simulink model "kestfilt_2048ch_60mhz"  (R2013b)
settings: Solver=FixedStepDiscrete  SolverMode=SingleTasking  StartTime=0.0  StopTime=100.0  FixedStep=0.1  RelTol=1e-3
undefined symbols (not defined in the file): calan_lib, comp_addsub, internal_oor, minmax, misc_lib, nonstop_vacc, pfb_coeff_gen_calc, seq_minmax, xlfda_numerator, xlipgetpartsetting
libraries: xbsIndex_r4 x3129, casper_library_misc x28, xps_library x27, dspsigops x16, casper_library_delays x7, simulink x2
(part 4 of 32)

== system kestfilt_2048ch_60mhz/dec_fir1 ==
  sync_in : Inport
  real1 : Inport  Port=2
  imag1 : Inport  Port=3
  real2 : Inport  Port=4
  imag2 : Inport  Port=5
  real3 : Inport  Port=6
  imag3 : Inport  Port=7
  real4 : Inport  Port=8
  imag4 : Inport  Port=9
  real5 : Inport  Port=10
  imag5 : Inport  Port=11
  real6 : Inport  Port=12
  imag6 : Inport  Port=13
  real7 : Inport  Port=14
  imag7 : Inport  Port=15
  real8 : Inport  Port=16
  imag8 : Inport  Port=17
  convert1 : xbsIndex_r4/Convert  gui_display_data_type=Fixed-point  arith_type="Signed  (2's comp)"  n_bits=8  bin_pt=7  float_type=Single  exp_bits=8  fraction_bits=24  quantization="Round  (unbiased: Even Values)"  overflow=Wrap  en=off  latency=2  dbl_ovrd=off  pipeline=off  block_type=convert
  convert2 : xbsIndex_r4/Convert  gui_display_data_type=Fixed-point  arith_type="Signed  (2's comp)"  n_bits=8  bin_pt=7  float_type=Single  exp_bits=8  fraction_bits=24  quantization="Round  (unbiased: Even Values)"  overflow=Wrap  en=off  latency=2  dbl_ovrd=off  pipeline=off  block_type=convert
  delay : xbsIndex_r4/Delay  rst=off  infoeditControl=Selection of Reset will increase slice count due to use of real FFs and instead of SRLs  en=off  latency=7  dbl_ovrd=off  reg_retiming=off  block_type=delay
  fir_col1 : Subsystem  AncestorBlock=casper_library_downconverter/fir_col  mask(fir_col){n_inputs=8, coeff=[0.00113   0.0022337   0.0028132   0.0028275   0.0023426   0.0015071   0.0005151  -0.0004352], add_latency=1, mult_latency=2, coeff_bit_width=25, coeff_bin_pt=24, first_stage_hdl=on, adder_imp=DSP48}
      mask prompts: n_inputs "Inputs"; coeff "Coefficients"; add_latency "Add latency"; mult_latency "Mult Latency"; coeff_bit_width "Coefficient bit width"; coeff_bin_pt "Coefficient binary point"; first_stage_hdl "Implement first stage of adder trees on output as behavioural HDL"; adder_imp "Adder implementation"
      mask init: same as kestfilt_2048ch_60mhz/dec_fir/fir_col1
      mask Help: eval('xlWeb(''http://casper.berkeley.edu/wiki/Fir_col'')')
      mask TypeOptions adder_imp: Behavioral | Fabric | DSP48
  fir_col10 : Subsystem  AncestorBlock=casper_library_downconverter/fir_col  mask(fir_col){n_inputs=8, coeff=[-0.0058263  -0.0086204   -0.010054  -0.0096853  -0.0073661   -0.003308   0.0019177   0.0074447], add_latency=1, mult_latency=2, coeff_bit_width=25, coeff_bin_pt=24, first_stage_hdl=on, adder_imp=DSP48}
      mask prompts: n_inputs "Inputs"; coeff "Coefficients"; add_latency "Add latency"; mult_latency "Mult Latency"; coeff_bit_width "Coefficient bit width"; coeff_bin_pt "Coefficient binary point"; first_stage_hdl "Implement first stage of adder trees on output as behavioural HDL"; adder_imp "Adder implementation"
      mask init: same as kestfilt_2048ch_60mhz/dec_fir/fir_col1
      mask Help: eval('xlWeb(''http://casper.berkeley.edu/wiki/Fir_col'')')
      mask TypeOptions adder_imp: Behavioral | Fabric | DSP48
  fir_col11 : Subsystem  AncestorBlock=casper_library_downconverter/fir_col  mask(fir_col){n_inputs=8, coeff=[0.0022453   0.0045072   0.0061467   0.0067686   0.0061328   0.0042185   0.0012532  -0.0023042], add_latency=1, mult_latency=2, coeff_bit_width=25, coeff_bin_pt=24, first_stage_hdl=on, adder_imp=DSP48}
      mask prompts: n_inputs "Inputs"; coeff "Coefficients"; add_latency "Add latency"; mult_latency "Mult Latency"; coeff_bit_width "Coefficient bit width"; coeff_bin_pt "Coefficient binary point"; first_stage_hdl "Implement first stage of adder trees on output as behavioural HDL"; adder_imp "Adder implementation"
      mask init: same as kestfilt_2048ch_60mhz/dec_fir/fir_col1
      mask Help: eval('xlWeb(''http://casper.berkeley.edu/wiki/Fir_col'')')
      mask TypeOptions adder_imp: Behavioral | Fabric | DSP48
  fir_col12 : Subsystem  AncestorBlock=casper_library_downconverter/fir_col  mask(fir_col){n_inputs=8, coeff=[-0.00034455  -0.0019414  -0.0033558  -0.0042822  -0.0044754  -0.0038077  -0.0023081 -0.00017465], add_latency=1, mult_latency=2, coeff_bit_width=25, coeff_bin_pt=24, first_stage_hdl=on, adder_imp=DSP48}
      mask prompts: n_inputs "Inputs"; coeff "Coefficients"; add_latency "Add latency"; mult_latency "Mult Latency"; coeff_bit_width "Coefficient bit width"; coeff_bin_pt "Coefficient binary point"; first_stage_hdl "Implement first stage of adder trees on output as behavioural HDL"; adder_imp "Adder implementation"
      mask init: same as kestfilt_2048ch_60mhz/dec_fir/fir_col1
      mask Help: eval('xlWeb(''http://casper.berkeley.edu/wiki/Fir_col'')')
      mask TypeOptions adder_imp: Behavioral | Fabric | DSP48
  fir_col13 : Subsystem  AncestorBlock=casper_library_downconverter/fir_col  mask(fir_col){n_inputs=8, coeff=[-0.0004352   0.0005151   0.0015071   0.0023426   0.0028275   0.0028132   0.0022337     0.00113], add_latency=1, mult_latency=2, coeff_bit_width=25, coeff_bin_pt=24, first_stage_hdl=on, adder_imp=DSP48}
      mask prompts: n_inputs "Inputs"; coeff "Coefficients"; add_latency "Add latency"; mult_latency "Mult Latency"; coeff_bit_width "Coefficient bit width"; coeff_bin_pt "Coefficient binary point"; first_stage_hdl "Implement first stage of adder trees on output as behavioural HDL"; adder_imp "Adder implementation"
      mask init: same as kestfilt_2048ch_60mhz/dec_fir/fir_col1
      mask Help: eval('xlWeb(''http://casper.berkeley.edu/wiki/Fir_col'')')
      mask TypeOptions adder_imp: Behavioral | Fabric | DSP48
  fir_col2 : Subsystem  AncestorBlock=casper_library_downconverter/fir_col  mask(fir_col){n_inputs=8, coeff=[-0.00017465  -0.0023081  -0.0038077  -0.0044754  -0.0042822  -0.0033558  -0.0019414 -0.00034455], add_latency=1, mult_latency=2, coeff_bit_width=25, coeff_bin_pt=24, first_stage_hdl=on, adder_imp=DSP48}
      mask prompts: n_inputs "Inputs"; coeff "Coefficients"; add_latency "Add latency"; mult_latency "Mult Latency"; coeff_bit_width "Coefficient bit width"; coeff_bin_pt "Coefficient binary point"; first_stage_hdl "Implement first stage of adder trees on output as behavioural HDL"; adder_imp "Adder implementation"
      mask init: same as kestfilt_2048ch_60mhz/dec_fir/fir_col1
      mask Help: eval('xlWeb(''http://casper.berkeley.edu/wiki/Fir_col'')')
      mask TypeOptions adder_imp: Behavioral | Fabric | DSP48
  fir_col3 : Subsystem  AncestorBlock=casper_library_downconverter/fir_col  mask(fir_col){n_inputs=8, coeff=[-0.0023042   0.0012532   0.0042185   0.0061328   0.0067686   0.0061467   0.0045072   0.0022453], add_latency=1, mult_latency=2, coeff_bit_width=25, coeff_bin_pt=24, first_stage_hdl=on, adder_imp=DSP48}
      mask prompts: n_inputs "Inputs"; coeff "Coefficients"; add_latency "Add latency"; mult_latency "Mult Latency"; coeff_bit_width "Coefficient bit width"; coeff_bin_pt "Coefficient binary point"; first_stage_hdl "Implement first stage of adder trees on output as behavioural HDL"; adder_imp "Adder implementation"
      mask init: same as kestfilt_2048ch_60mhz/dec_fir/fir_col1
      mask Help: eval('xlWeb(''http://casper.berkeley.edu/wiki/Fir_col'')')
      mask TypeOptions adder_imp: Behavioral | Fabric | DSP48
  fir_col4 : Subsystem  AncestorBlock=casper_library_downconverter/fir_col  mask(fir_col){n_inputs=8, coeff=[0.0074447   0.0019177   -0.003308  -0.0073661  -0.0096853   -0.010054  -0.0086204  -0.0058263], add_latency=1, mult_latency=2, coeff_bit_width=25, coeff_bin_pt=24, first_stage_hdl=on, adder_imp=DSP48}
      mask prompts: n_inputs "Inputs"; coeff "Coefficients"; add_latency "Add latency"; mult_latency "Mult Latency"; coeff_bit_width "Coefficient bit width"; coeff_bin_pt "Coefficient binary point"; first_stage_hdl "Implement first stage of adder trees on output as behavioural HDL"; adder_imp "Adder implementation"
      mask init: same as kestfilt_2048ch_60mhz/dec_fir/fir_col1
      mask Help: eval('xlWeb(''http://casper.berkeley.edu/wiki/Fir_col'')')
      mask TypeOptions adder_imp: Behavioral | Fabric | DSP48
  fir_col5 : Subsystem  AncestorBlock=casper_library_downconverter/fir_col  mask(fir_col){n_inputs=8, coeff=[-0.018838  -0.0098708 -0.00058855   0.0074448     0.01308    0.015703     0.01527    0.012239], add_latency=1, mult_latency=2, coeff_bit_width=25, coeff_bin_pt=24, first_stage_hdl=on, adder_imp=DSP48}
      mask prompts: n_inputs "Inputs"; coeff "Coefficients"; add_latency "Add latency"; mult_latency "Mult Latency"; coeff_bit_width "Coefficient bit width"; coeff_bin_pt "Coefficient binary point"; first_stage_hdl "Implement first stage of adder trees on output as behavioural HDL"; adder_imp "Adder implementation"
      mask init: same as kestfilt_2048ch_60mhz/dec_fir/fir_col1
      mask Help: eval('xlWeb(''http://casper.berkeley.edu/wiki/Fir_col'')')
      mask TypeOptions adder_imp: Behavioral | Fabric | DSP48
  fir_col6 : Subsystem  AncestorBlock=casper_library_downconverter/fir_col  mask(fir_col){n_inputs=8, coeff=[0.065516    0.039865    0.016011  -0.0038951   -0.018338   -0.026596   -0.028772   -0.025715], add_latency=1, mult_latency=2, coeff_bit_width=25, coeff_bin_pt=24, first_stage_hdl=on, adder_imp=DSP48}
      mask prompts: n_inputs "Inputs"; coeff "Coefficients"; add_latency "Add latency"; mult_latency "Mult Latency"; coeff_bit_width "Coefficient bit width"; coeff_bin_pt "Coefficient binary point"; first_stage_hdl "Implement first stage of adder trees on output as behavioural HDL"; adder_imp "Adder implementation"
      mask init: same as kestfilt_2048ch_60mhz/dec_fir/fir_col1
      mask Help: eval('xlWeb(''http://casper.berkeley.edu/wiki/Fir_col'')')
      mask TypeOptions adder_imp: Behavioral | Fabric | DSP48
  fir_col7 : Subsystem  AncestorBlock=casper_library_downconverter/fir_col  mask(fir_col){n_inputs=8, coeff=[0.090423     0.11197     0.12783     0.13623     0.13623     0.12783     0.11197    0.090423], add_latency=1, mult_latency=2, coeff_bit_width=25, coeff_bin_pt=24, first_stage_hdl=on, adder_imp=DSP48}
      mask prompts: n_inputs "Inputs"; coeff "Coefficients"; add_latency "Add latency"; mult_latency "Mult Latency"; coeff_bit_width "Coefficient bit width"; coeff_bin_pt "Coefficient binary point"; first_stage_hdl "Implement first stage of adder trees on output as behavioural HDL"; adder_imp "Adder implementation"
      mask init: same as kestfilt_2048ch_60mhz/dec_fir/fir_col1
      mask Help: eval('xlWeb(''http://casper.berkeley.edu/wiki/Fir_col'')')
      mask TypeOptions adder_imp: Behavioral | Fabric | DSP48
  fir_col8 : Subsystem  AncestorBlock=casper_library_downconverter/fir_col  mask(fir_col){n_inputs=8, coeff=[-0.025715   -0.028772   -0.026596   -0.018338  -0.0038951    0.016011    0.039865    0.065516], add_latency=1, mult_latency=2, coeff_bit_width=25, coeff_bin_pt=24, first_stage_hdl=on, adder_imp=DSP48}
      mask prompts: n_inputs "Inputs"; coeff "Coefficients"; add_latency "Add latency"; mult_latency "Mult Latency"; coeff_bit_width "Coefficient bit width"; coeff_bin_pt "Coefficient binary point"; first_stage_hdl "Implement first stage of adder trees on output as behavioural HDL"; adder_imp "Adder implementation"
      mask init: same as kestfilt_2048ch_60mhz/dec_fir/fir_col1
      mask Help: eval('xlWeb(''http://casper.berkeley.edu/wiki/Fir_col'')')
      mask TypeOptions adder_imp: Behavioral | Fabric | DSP48
  fir_col9 : Subsystem  AncestorBlock=casper_library_downconverter/fir_col  mask(fir_col){n_inputs=8, coeff=[0.012239     0.01527    0.015703     0.01308   0.0074448 -0.00058855  -0.0098708   -0.018838], add_latency=1, mult_latency=2, coeff_bit_width=25, coeff_bin_pt=24, first_stage_hdl=on, adder_imp=DSP48}
      mask prompts: n_inputs "Inputs"; coeff "Coefficients"; add_latency "Add latency"; mult_latency "Mult Latency"; coeff_bit_width "Coefficient bit width"; coeff_bin_pt "Coefficient binary point"; first_stage_hdl "Implement first stage of adder trees on output as behavioural HDL"; adder_imp "Adder implementation"
      mask init: same as kestfilt_2048ch_60mhz/dec_fir/fir_col1
      mask Help: eval('xlWeb(''http://casper.berkeley.edu/wiki/Fir_col'')')
      mask TypeOptions adder_imp: Behavioral | Fabric | DSP48
  imag_sum : Subsystem  AncestorBlock=casper_library_misc/adder_tree  mask(adder_tree){n_inputs=13, latency=1, adder_imp=DSP48, first_stage_hdl=off}
      mask prompts: n_inputs "Number of Inputs"; latency "Add Latency"; adder_imp "Adder implementation"; first_stage_hdl "Use behavioural HDL for first stage of adders"
      mask help:
      | Sums all inputs using a tree of adds and delays.
      |
      | Number of inputs: The number of inputs to the block to be summed
      | Add latency: The number of clock cycles to perform one addition (affects timing)..
      | Adder implementation: choice of fabric or DSP48E core, or behavioral HDL
      | Use behavioural HDL for first stage of adders: Causes the first stage of adders to be absorbed into DSP blocks if multipliers precede them (Virtex 5). Overrides Adder implementation
      mask init:
      | adder_tree_init(gcb, ...
      |     'n_inputs', n_inputs, ...
      |     'latency', latency, ...
      |     'adder_imp', adder_imp, ...
      |     'first_stage_hdl', first_stage_hdl);
      settings: AttributesFormatString=latency 4
      mask Help: eval('xlWeb(''http://casper.berkeley.edu/wiki/Adder_tree'')')
      mask TypeOptions adder_imp: Behavioral | Fabric | DSP48
  real_sum : Subsystem  AncestorBlock=casper_library_misc/adder_tree  mask(adder_tree){n_inputs=13, latency=1, adder_imp=DSP48, first_stage_hdl=off}
      mask prompts: n_inputs "Number of Inputs"; latency "Add Latency"; adder_imp "Adder implementation"; first_stage_hdl "Use behavioural HDL for first stage of adders"
      mask help:
      | Sums all inputs using a tree of adds and delays.
      |
      | Number of inputs: The number of inputs to the block to be summed
      | Add latency: The number of clock cycles to perform one addition (affects timing)..
      | Adder implementation: choice of fabric or DSP48E core, or behavioral HDL
      | Use behavioural HDL for first stage of adders: Causes the first stage of adders to be absorbed into DSP blocks if multipliers precede them (Virtex 5). Overrides Adder implementation
      mask init:
      | adder_tree_init(gcb, ...
      |     'n_inputs', n_inputs, ...
      |     'latency', latency, ...
      |     'adder_imp', adder_imp, ...
      |     'first_stage_hdl', first_stage_hdl);
      settings: AttributesFormatString=latency 4
      mask Help: eval('xlWeb(''http://casper.berkeley.edu/wiki/Adder_tree'')')
      mask TypeOptions adder_imp: Behavioral | Fabric | DSP48
  ri_to_c : casper_library_misc/ri_to_c
  shift1 : xbsIndex_r4/Shift  shift_dir=Left  shift_bits=1  en=off  latency=0  precision=Full  arith_type="Signed  (2's comp)"  n_bits=16  bin_pt=14  quantization=Truncate  overflow=Wrap  dbl_ovrd=off  block_type=shift
  shift2 : xbsIndex_r4/Shift  shift_dir=Left  shift_bits=1  en=off  latency=0  precision=Full  arith_type="Signed  (2's comp)"  n_bits=16  bin_pt=14  quantization=Truncate  overflow=Wrap  dbl_ovrd=off  block_type=shift
  sync_out : Outport
  dout : Outport  Port=2
  wires:
  real1/1 -> fir_col1/1(real1)
  imag1/1 -> fir_col1/2(imag1)
  real2/1 -> fir_col1/3(real2)
  imag2/1 -> fir_col1/4(imag2)
  real3/1 -> fir_col1/5(real3)
  imag3/1 -> fir_col1/6(imag3)
  real4/1 -> fir_col1/7(real4)
  imag4/1 -> fir_col1/8(imag4)
  real5/1 -> fir_col1/9(real5)
  imag5/1 -> fir_col1/10(imag5)
  real6/1 -> fir_col1/11(real6)
  imag6/1 -> fir_col1/12(imag6)
  real7/1 -> fir_col1/13(real7)
  imag7/1 -> fir_col1/14(imag7)
  real8/1 -> fir_col1/15(real8)
  imag8/1 -> fir_col1/16(imag8)
  fir_col1/17(real_sum) -> real_sum/2(din1)
  fir_col1/18(imag_sum) -> imag_sum/2(din1)
  fir_col1/1(real_out1) -> fir_col2/1(real1)
  fir_col1/2(imag_out1) -> fir_col2/2(imag1)
  fir_col1/3(real_out2) -> fir_col2/3(real2)
  fir_col1/4(imag_out2) -> fir_col2/4(imag2)
  fir_col1/5(real_out3) -> fir_col2/5(real3)
  fir_col1/6(imag_out3) -> fir_col2/6(imag3)
  fir_col1/7(real_out4) -> fir_col2/7(real4)
  fir_col1/8(imag_out4) -> fir_col2/8(imag4)
  fir_col1/9(real_out5) -> fir_col2/9(real5)
  fir_col1/10(imag_out5) -> fir_col2/10(imag5)
  fir_col1/11(real_out6) -> fir_col2/11(real6)
  fir_col1/12(imag_out6) -> fir_col2/12(imag6)
  fir_col1/13(real_out7) -> fir_col2/13(real7)
  fir_col1/14(imag_out7) -> fir_col2/14(imag7)
  fir_col1/15(real_out8) -> fir_col2/15(real8)
  fir_col1/16(imag_out8) -> fir_col2/16(imag8)
  fir_col2/17(real_sum) -> real_sum/3(din2)
  fir_col2/18(imag_sum) -> imag_sum/3(din2)
  fir_col2/1(real_out1) -> fir_col3/1(real1)
  fir_col2/2(imag_out1) -> fir_col3/2(imag1)
  fir_col2/3(real_out2) -> fir_col3/3(real2)
  fir_col2/4(imag_out2) -> fir_col3/4(imag2)
  fir_col2/5(real_out3) -> fir_col3/5(real3)
  fir_col2/6(imag_out3) -> fir_col3/6(imag3)
  fir_col2/7(real_out4) -> fir_col3/7(real4)
  fir_col2/8(imag_out4) -> fir_col3/8(imag4)
  fir_col2/9(real_out5) -> fir_col3/9(real5)
  fir_col2/10(imag_out5) -> fir_col3/10(imag5)
  fir_col2/11(real_out6) -> fir_col3/11(real6)
  fir_col2/12(imag_out6) -> fir_col3/12(imag6)
  fir_col2/13(real_out7) -> fir_col3/13(real7)
  fir_col2/14(imag_out7) -> fir_col3/14(imag7)
  fir_col2/15(real_out8) -> fir_col3/15(real8)
  fir_col2/16(imag_out8) -> fir_col3/16(imag8)
  fir_col3/17(real_sum) -> real_sum/4(din3)
  fir_col3/18(imag_sum) -> imag_sum/4(din3)
  fir_col3/1(real_out1) -> fir_col4/1(real1)
  fir_col3/2(imag_out1) -> fir_col4/2(imag1)
  fir_col3/3(real_out2) -> fir_col4/3(real2)
  fir_col3/4(imag_out2) -> fir_col4/4(imag2)
  fir_col3/5(real_out3) -> fir_col4/5(real3)
  fir_col3/6(imag_out3) -> fir_col4/6(imag3)
  fir_col3/7(real_out4) -> fir_col4/7(real4)
  fir_col3/8(imag_out4) -> fir_col4/8(imag4)
  fir_col3/9(real_out5) -> fir_col4/9(real5)
  fir_col3/10(imag_out5) -> fir_col4/10(imag5)
  fir_col3/11(real_out6) -> fir_col4/11(real6)
  fir_col3/12(imag_out6) -> fir_col4/12(imag6)
  fir_col3/13(real_out7) -> fir_col4/13(real7)
  fir_col3/14(imag_out7) -> fir_col4/14(imag7)
  fir_col3/15(real_out8) -> fir_col4/15(real8)
  fir_col3/16(imag_out8) -> fir_col4/16(imag8)
  fir_col4/17(real_sum) -> real_sum/5(din4)
  fir_col4/18(imag_sum) -> imag_sum/5(din4)
  fir_col4/1(real_out1) -> fir_col5/1(real1)
  fir_col4/2(imag_out1) -> fir_col5/2(imag1)
  fir_col4/3(real_out2) -> fir_col5/3(real2)
  fir_col4/4(imag_out2) -> fir_col5/4(imag2)
  fir_col4/5(real_out3) -> fir_col5/5(real3)
  fir_col4/6(imag_out3) -> fir_col5/6(imag3)
  fir_col4/7(real_out4) -> fir_col5/7(real4)
  fir_col4/8(imag_out4) -> fir_col5/8(imag4)
  fir_col4/9(real_out5) -> fir_col5/9(real5)
  fir_col4/10(imag_out5) -> fir_col5/10(imag5)
  fir_col4/11(real_out6) -> fir_col5/11(real6)
  fir_col4/12(imag_out6) -> fir_col5/12(imag6)
  fir_col4/13(real_out7) -> fir_col5/13(real7)
  fir_col4/14(imag_out7) -> fir_col5/14(imag7)
  fir_col4/15(real_out8) -> fir_col5/15(real8)
  fir_col4/16(imag_out8) -> fir_col5/16(imag8)
  fir_col5/17(real_sum) -> real_sum/6(din5)
  fir_col5/18(imag_sum) -> imag_sum/6(din5)
  fir_col5/1(real_out1) -> fir_col6/1(real1)
  fir_col5/2(imag_out1) -> fir_col6/2(imag1)
  fir_col5/3(real_out2) -> fir_col6/3(real2)
  fir_col5/4(imag_out2) -> fir_col6/4(imag2)
  fir_col5/5(real_out3) -> fir_col6/5(real3)
  fir_col5/6(imag_out3) -> fir_col6/6(imag3)
  fir_col5/7(real_out4) -> fir_col6/7(real4)
  fir_col5/8(imag_out4) -> fir_col6/8(imag4)
  fir_col5/9(real_out5) -> fir_col6/9(real5)
  fir_col5/10(imag_out5) -> fir_col6/10(imag5)
  fir_col5/11(real_out6) -> fir_col6/11(real6)
  fir_col5/12(imag_out6) -> fir_col6/12(imag6)
  fir_col5/13(real_out7) -> fir_col6/13(real7)
  fir_col5/14(imag_out7) -> fir_col6/14(imag7)
  fir_col5/15(real_out8) -> fir_col6/15(real8)
  fir_col5/16(imag_out8) -> fir_col6/16(imag8)
  fir_col6/17(real_sum) -> real_sum/7(din6)
  fir_col6/18(imag_sum) -> imag_sum/7(din6)
  fir_col6/1(real_out1) -> fir_col7/1(real1)
  fir_col6/2(imag_out1) -> fir_col7/2(imag1)
  fir_col6/3(real_out2) -> fir_col7/3(real2)
  fir_col6/4(imag_out2) -> fir_col7/4(imag2)
  fir_col6/5(real_out3) -> fir_col7/5(real3)
  fir_col6/6(imag_out3) -> fir_col7/6(imag3)
  fir_col6/7(real_out4) -> fir_col7/7(real4)
  fir_col6/8(imag_out4) -> fir_col7/8(imag4)
  fir_col6/9(real_out5) -> fir_col7/9(real5)
  fir_col6/10(imag_out5) -> fir_col7/10(imag5)
  fir_col6/11(real_out6) -> fir_col7/11(real6)
  fir_col6/12(imag_out6) -> fir_col7/12(imag6)
  fir_col6/13(real_out7) -> fir_col7/13(real7)
  fir_col6/14(imag_out7) -> fir_col7/14(imag7)
  fir_col6/15(real_out8) -> fir_col7/15(real8)
  fir_col6/16(imag_out8) -> fir_col7/16(imag8)
  fir_col7/17(real_sum) -> real_sum/8(din7)
  fir_col7/18(imag_sum) -> imag_sum/8(din7)
  fir_col7/1(real_out1) -> fir_col8/1(real1)
  fir_col7/2(imag_out1) -> fir_col8/2(imag1)
  fir_col7/3(real_out2) -> fir_col8/3(real2)
  fir_col7/4(imag_out2) -> fir_col8/4(imag2)
  fir_col7/5(real_out3) -> fir_col8/5(real3)
  fir_col7/6(imag_out3) -> fir_col8/6(imag3)
  fir_col7/7(real_out4) -> fir_col8/7(real4)
  fir_col7/8(imag_out4) -> fir_col8/8(imag4)
  fir_col7/9(real_out5) -> fir_col8/9(real5)
  fir_col7/10(imag_out5) -> fir_col8/10(imag5)
  fir_col7/11(real_out6) -> fir_col8/11(real6)
  fir_col7/12(imag_out6) -> fir_col8/12(imag6)
  fir_col7/13(real_out7) -> fir_col8/13(real7)
  fir_col7/14(imag_out7) -> fir_col8/14(imag7)
  fir_col7/15(real_out8) -> fir_col8/15(real8)
  fir_col7/16(imag_out8) -> fir_col8/16(imag8)
  fir_col8/17(real_sum) -> real_sum/9(din8)
  fir_col8/18(imag_sum) -> imag_sum/9(din8)
  fir_col8/1(real_out1) -> fir_col9/1(real1)
  fir_col8/2(imag_out1) -> fir_col9/2(imag1)
  fir_col8/3(real_out2) -> fir_col9/3(real2)
  fir_col8/4(imag_out2) -> fir_col9/4(imag2)
  fir_col8/5(real_out3) -> fir_col9/5(real3)
  fir_col8/6(imag_out3) -> fir_col9/6(imag3)
  fir_col8/7(real_out4) -> fir_col9/7(real4)
  fir_col8/8(imag_out4) -> fir_col9/8(imag4)
  fir_col8/9(real_out5) -> fir_col9/9(real5)
  fir_col8/10(imag_out5) -> fir_col9/10(imag5)
  fir_col8/11(real_out6) -> fir_col9/11(real6)
  fir_col8/12(imag_out6) -> fir_col9/12(imag6)
  fir_col8/13(real_out7) -> fir_col9/13(real7)
  fir_col8/14(imag_out7) -> fir_col9/14(imag7)
  fir_col8/15(real_out8) -> fir_col9/15(real8)
  fir_col8/16(imag_out8) -> fir_col9/16(imag8)
  fir_col9/17(real_sum) -> real_sum/10(din9)
  fir_col9/18(imag_sum) -> imag_sum/10(din9)
  fir_col9/1(real_out1) -> fir_col10/1(real1)
  fir_col9/2(imag_out1) -> fir_col10/2(imag1)
  fir_col9/3(real_out2) -> fir_col10/3(real2)
  fir_col9/4(imag_out2) -> fir_col10/4(imag2)
  fir_col9/5(real_out3) -> fir_col10/5(real3)
  fir_col9/6(imag_out3) -> fir_col10/6(imag3)
  fir_col9/7(real_out4) -> fir_col10/7(real4)
  fir_col9/8(imag_out4) -> fir_col10/8(imag4)
  fir_col9/9(real_out5) -> fir_col10/9(real5)
  fir_col9/10(imag_out5) -> fir_col10/10(imag5)
  fir_col9/11(real_out6) -> fir_col10/11(real6)
  fir_col9/12(imag_out6) -> fir_col10/12(imag6)
  fir_col9/13(real_out7) -> fir_col10/13(real7)
  fir_col9/14(imag_out7) -> fir_col10/14(imag7)
  fir_col9/15(real_out8) -> fir_col10/15(real8)
  fir_col9/16(imag_out8) -> fir_col10/16(imag8)
  fir_col10/17(real_sum) -> real_sum/11(din10)
  fir_col10/18(imag_sum) -> imag_sum/11(din10)
  fir_col10/1(real_out1) -> fir_col11/1(real1)
  fir_col10/2(imag_out1) -> fir_col11/2(imag1)
  fir_col10/3(real_out2) -> fir_col11/3(real2)
  fir_col10/4(imag_out2) -> fir_col11/4(imag2)
  fir_col10/5(real_out3) -> fir_col11/5(real3)
  fir_col10/6(imag_out3) -> fir_col11/6(imag3)
  fir_col10/7(real_out4) -> fir_col11/7(real4)
  fir_col10/8(imag_out4) -> fir_col11/8(imag4)
  fir_col10/9(real_out5) -> fir_col11/9(real5)
  fir_col10/10(imag_out5) -> fir_col11/10(imag5)
  fir_col10/11(real_out6) -> fir_col11/11(real6)
  fir_col10/12(imag_out6) -> fir_col11/12(imag6)
  fir_col10/13(real_out7) -> fir_col11/13(real7)
  fir_col10/14(imag_out7) -> fir_col11/14(imag7)
  fir_col10/15(real_out8) -> fir_col11/15(real8)
  fir_col10/16(imag_out8) -> fir_col11/16(imag8)
  fir_col11/17(real_sum) -> real_sum/12(din11)
  fir_col11/18(imag_sum) -> imag_sum/12(din11)
  fir_col11/1(real_out1) -> fir_col12/1(real1)
  fir_col11/2(imag_out1) -> fir_col12/2(imag1)
  fir_col11/3(real_out2) -> fir_col12/3(real2)
  fir_col11/4(imag_out2) -> fir_col12/4(imag2)
  fir_col11/5(real_out3) -> fir_col12/5(real3)
  fir_col11/6(imag_out3) -> fir_col12/6(imag3)
  fir_col11/7(real_out4) -> fir_col12/7(real4)
  fir_col11/8(imag_out4) -> fir_col12/8(imag4)
  fir_col11/9(real_out5) -> fir_col12/9(real5)
  fir_col11/10(imag_out5) -> fir_col12/10(imag5)
  fir_col11/11(real_out6) -> fir_col12/11(real6)
  fir_col11/12(imag_out6) -> fir_col12/12(imag6)
  fir_col11/13(real_out7) -> fir_col12/13(real7)
  fir_col11/14(imag_out7) -> fir_col12/14(imag7)
  fir_col11/15(real_out8) -> fir_col12/15(real8)
  fir_col11/16(imag_out8) -> fir_col12/16(imag8)
  fir_col12/17(real_sum) -> real_sum/13(din12)
  fir_col12/18(imag_sum) -> imag_sum/13(din12)
  fir_col12/1(real_out1) -> fir_col13/1(real1)
  fir_col12/2(imag_out1) -> fir_col13/2(imag1)
  fir_col12/3(real_out2) -> fir_col13/3(real2)
  fir_col12/4(imag_out2) -> fir_col13/4(imag2)
  fir_col12/5(real_out3) -> fir_col13/5(real3)
  fir_col12/6(imag_out3) -> fir_col13/6(imag3)
  fir_col12/7(real_out4) -> fir_col13/7(real4)
  fir_col12/8(imag_out4) -> fir_col13/8(imag4)
  fir_col12/9(real_out5) -> fir_col13/9(real5)
  fir_col12/10(imag_out5) -> fir_col13/10(imag5)
  fir_col12/11(real_out6) -> fir_col13/11(real6)
  fir_col12/12(imag_out6) -> fir_col13/12(imag6)
  fir_col12/13(real_out7) -> fir_col13/13(real7)
  fir_col12/14(imag_out7) -> fir_col13/14(imag7)
  fir_col12/15(real_out8) -> fir_col13/15(real8)
  fir_col12/16(imag_out8) -> fir_col13/16(imag8)
  fir_col13/17(real_sum) -> real_sum/14(din13)
  fir_col13/18(imag_sum) -> imag_sum/14(din13)
  real_sum/2(dout) -> shift1/1
  imag_sum/2(dout) -> shift2/1
  shift1/1 -> convert1/1
  shift2/1 -> convert2/1
  convert1/1 -> ri_to_c/1
  convert2/1 -> ri_to_c/2
  ri_to_c/1 -> dout/1
  sync_in/1 -> delay/1
  delay/1 -> real_sum/1(sync), imag_sum/1(sync)
  real_sum/1(sync_out) -> sync_out/1

== system kestfilt_2048ch_60mhz/dout0_0 ==
  addr : Inport
  data_in : Inport  Port=2
  we : Inport  Port=3
  calc_add : Subsystem  mask{data_width=64, addr_width=11, sample_rate=sample_rate}
      mask prompts: data_width "data width"; addr_width "address width"; sample_rate "sample rate"
  convert_addr : xbsIndex_r4/Convert  gui_display_data_type=Fixed-point  arith_type=Unsigned  n_bits=addr_width  bin_pt=0  float_type=Single  exp_bits=8  fraction_bits=24  quantization=Truncate  overflow=Wrap  en=off  latency=0  dbl_ovrd=off  pipeline=off  block_type=convert
      settings: xl_area=[0, 0, 0, 0, 0, 0, 0]
  convert_din1 : xbsIndex_r4/Convert  gui_display_data_type=Fixed-point  arith_type=Unsigned  n_bits=64  bin_pt=0  float_type=Single  exp_bits=8  fraction_bits=24  quantization=Truncate  overflow=Wrap  en=off  latency=0  dbl_ovrd=off  pipeline=off  block_type=convert
      settings: xl_area=[0, 0, 0, 0, 0, 0, 0]
  convert_we : xbsIndex_r4/Convert  gui_display_data_type=Fixed-point  arith_type=Unsigned  n_bits=1  bin_pt=0  float_type=Single  exp_bits=8  fraction_bits=24  quantization=Truncate  overflow=Wrap  en=off  latency=0  dbl_ovrd=off  pipeline=off  block_type=convert
      settings: xl_area=[0, 0, 0, 0, 0, 0, 0]
  kestfilt_2048ch_60mhz_dout0_0_addr : xbsIndex_r4/Gateway Out  inherit_from_input=off  hdl_port=on  timing_constraint=None  locs_specified=off  LOCs={'A5','B9','A9','C1','A3','G6','E9','A6','A7','A8','B8','B1','B3','D9','B5','B4','B6','C2'}  UseAsDAC=off  DACChannel='1'  block_type=gatewayout
      settings: infoedit="Gateway out block.  Converts Xilinx fixed point inputs into ouputs of type Simulink integer, double, or fixed point.<P><P>Hardware notes:  In hardware these blocks become top level output ports or are discarded, depending on how they are configured."  xl_area=[0, 0, 0, 0, 0, 0, 0]  sginterface={'Nallatech'=>{'xdspkit'=>{'non_memory_mapped_port'=>'uprev_Shared_BRAM_addr'}},'Xilinx'=>{'jtaghwcosim'=>{'non_memory_mapped_port'=>'uprev_Shared_BRAM_addr'},'xdspkit'=>{'non_memory_mapped_port'=>'uprev_Shared_BRAM_addr'}}}
  kestfilt_2048ch_60mhz_dout0_0_data_in : xbsIndex_r4/Gateway Out  inherit_from_input=off  hdl_port=on  timing_constraint=None  locs_specified=off  LOCs={'B21','B22','A22','B23','B19','C19','A20','A21','A23','B24','A24','A25','E18','D18','C18','B18'}  UseAsDAC=off  DACChannel='1'  block_type=gatewayout
      settings: infoedit="Gateway out block.  Converts Xilinx fixed point inputs into ouputs of type Simulink integer, double, or fixed point.<P><P>Hardware notes:  In hardware these blocks become top level output ports or are discarded, depending on how they are configured."  xl_area=[0, 0, 0, 0, 0, 0, 0]  sginterface={'Nallatech'=>{'xdspkit'=>{'non_memory_mapped_port'=>'uprev_Shared_BRAM_data_in'}},'Xilinx'=>{'jtaghwcosim'=>{'non_memory_mapped_port'=>'uprev_Shared_BRAM_data_in'},'xdspkit'=>{'non_memory_mapped_port'=>'uprev_Shared_BRAM_data_in'}}}
  kestfilt_2048ch_60mhz_dout0_0_data_out : xbsIndex_r4/Gateway In  gui_display_data_type=Fixed-point  arith_type=Unsigned  n_bits=64  bin_pt=0  preci_type=Single  exp_width=8  frac_width=24  quantization=Truncate  overflow=Wrap  period=sample_rate  dbl_ovrd=off  timing_constraint=None  locs_specified=off  LOCs={}  UseAsADC=off  ADCChannel='1'  inherit_from_input=off  hdl_port=on  block_type=gatewayin
      settings: xl_area=[0, 0, 0, 0, 0, 0, 0]
  kestfilt_2048ch_60mhz_dout0_0_we : xbsIndex_r4/Gateway Out  inherit_from_input=off  hdl_port=on  timing_constraint=None  locs_specified=off  LOCs={'A14'}  UseAsDAC=off  DACChannel='1'  block_type=gatewayout
      settings: infoedit="Gateway out block.  Converts Xilinx fixed point inputs into ouputs of type Simulink integer, double, or fixed point.<P><P>Hardware notes:  In hardware these blocks become top level output ports or are discarded, depending on how they are configured."  xl_area=[0, 0, 0, 0, 0, 0, 0]
  mem : Subsystem
  munge_in : Subsystem  AncestorBlock=casper_library_flow_control/munge  mask(munge){divisions=2, div_size=[32 32], order=[1  0], arith_type_out=Unsigned, bin_pt_out=0}
      mask prompts: divisions "Number of divisions"; div_size "Division size (bits)"; order "Division packing order"; arith_type_out "Output arithmetic type"; bin_pt_out "Output binary point"
      mask help: Splits an input bus into the specified number of divisions and then recombines them in the order specified (most significant division = 0,least = number divisions-1)
      mask init:
      | munge_init(gcb, ...
      |     'divisions', divisions, ...
      |     'div_size', div_size, ...
      |     'order', order, ...
      |     'arith_type_out', arith_type_out, ...
      |     'bin_pt_out', bin_pt_out);
      settings: AttributesFormatString=|
      | split:[32 32]
      | join:[1 0]
      | Unsigned [64,0]
      mask TypeOptions arith_type_out: Unsigned | Signed  (2's comp) | Floating-point
  munge_out : Subsystem  AncestorBlock=casper_library_flow_control/munge  mask(munge){divisions=2, div_size=[32 32], order=[1  0], arith_type_out=Unsigned, bin_pt_out=0}
      mask prompts: divisions "Number of divisions"; div_size "Division size (bits)"; order "Division packing order"; arith_type_out "Output arithmetic type"; bin_pt_out "Output binary point"
      mask help: Splits an input bus into the specified number of divisions and then recombines them in the order specified (most significant division = 0,least = number divisions-1)
      mask init:
      | munge_init(gcb, ...
      |     'divisions', divisions, ...
      |     'div_size', div_size, ...
      |     'order', order, ...
      |     'arith_type_out', arith_type_out, ...
      |     'bin_pt_out', bin_pt_out);
      settings: AttributesFormatString=|
      | split:[32 32]
      | join:[1 0]
      | Unsigned [64,0]
      mask TypeOptions arith_type_out: Unsigned | Signed  (2's comp) | Floating-point
  data_out : Outport
  wires:
  munge_in/1(dout) -> convert_din1/1
  munge_out/1(dout) -> data_out/1
  we/1 -> convert_we/1
  addr/1 -> calc_add/1(in)
  mem/1(Out1) -> kestfilt_2048ch_60mhz_dout0_0_data_out/1
  kestfilt_2048ch_60mhz_dout0_0_data_out/1 -> munge_out/1(din)
  convert_we/1 -> kestfilt_2048ch_60mhz_dout0_0_we/1
  kestfilt_2048ch_60mhz_dout0_0_addr/1 -> mem/1(In1)
  kestfilt_2048ch_60mhz_dout0_0_data_in/1 -> mem/2(In2)
  kestfilt_2048ch_60mhz_dout0_0_we/1 -> mem/3(In3)
  calc_add/1(out) -> convert_addr/1
  data_in/1 -> munge_in/1(din)
  convert_din1/1 -> kestfilt_2048ch_60mhz_dout0_0_data_in/1
  convert_addr/1 -> kestfilt_2048ch_60mhz_dout0_0_addr/1

== system kestfilt_2048ch_60mhz/dout1_0 ==
  addr : Inport
  data_in : Inport  Port=2
  we : Inport  Port=3
  calc_add : Subsystem  mask{data_width=64, addr_width=11, sample_rate=sample_rate}
      mask prompts: data_width "data width"; addr_width "address width"; sample_rate "sample rate"
  convert_addr : xbsIndex_r4/Convert  gui_display_data_type=Fixed-point  arith_type=Unsigned  n_bits=addr_width  bin_pt=0  float_type=Single  exp_bits=8  fraction_bits=24  quantization=Truncate  overflow=Wrap  en=off  latency=0  dbl_ovrd=off  pipeline=off  block_type=convert
      settings: xl_area=[0, 0, 0, 0, 0, 0, 0]
  convert_din1 : xbsIndex_r4/Convert  gui_display_data_type=Fixed-point  arith_type=Unsigned  n_bits=64  bin_pt=0  float_type=Single  exp_bits=8  fraction_bits=24  quantization=Truncate  overflow=Wrap  en=off  latency=0  dbl_ovrd=off  pipeline=off  block_type=convert
      settings: xl_area=[0, 0, 0, 0, 0, 0, 0]
  convert_we : xbsIndex_r4/Convert  gui_display_data_type=Fixed-point  arith_type=Unsigned  n_bits=1  bin_pt=0  float_type=Single  exp_bits=8  fraction_bits=24  quantization=Truncate  overflow=Wrap  en=off  latency=0  dbl_ovrd=off  pipeline=off  block_type=convert
      settings: xl_area=[0, 0, 0, 0, 0, 0, 0]
  kestfilt_60mhz_nyq2_dout1_0_addr : xbsIndex_r4/Gateway Out  inherit_from_input=off  hdl_port=on  timing_constraint=None  locs_specified=off  LOCs={'A5','B9','A9','C1','A3','G6','E9','A6','A7','A8','B8','B1','B3','D9','B5','B4','B6','C2'}  UseAsDAC=off  DACChannel='1'  block_type=gatewayout
      settings: infoedit="Gateway out block.  Converts Xilinx fixed point inputs into ouputs of type Simulink integer, double, or fixed point.<P><P>Hardware notes:  In hardware these blocks become top level output ports or are discarded, depending on how they are configured."  xl_area=[0, 0, 0, 0, 0, 0, 0]  sginterface={'Nallatech'=>{'xdspkit'=>{'non_memory_mapped_port'=>'uprev_Shared_BRAM_addr'}},'Xilinx'=>{'jtaghwcosim'=>{'non_memory_mapped_port'=>'uprev_Shared_BRAM_addr'},'xdspkit'=>{'non_memory_mapped_port'=>'uprev_Shared_BRAM_addr'}}}
  kestfilt_60mhz_nyq2_dout1_0_data_in : xbsIndex_r4/Gateway Out  inherit_from_input=off  hdl_port=on  timing_constraint=None  locs_specified=off  LOCs={'B21','B22','A22','B23','B19','C19','A20','A21','A23','B24','A24','A25','E18','D18','C18','B18'}  UseAsDAC=off  DACChannel='1'  block_type=gatewayout
      settings: infoedit="Gateway out block.  Converts Xilinx fixed point inputs into ouputs of type Simulink integer, double, or fixed point.<P><P>Hardware notes:  In hardware these blocks become top level output ports or are discarded, depending on how they are configured."  xl_area=[0, 0, 0, 0, 0, 0, 0]  sginterface={'Nallatech'=>{'xdspkit'=>{'non_memory_mapped_port'=>'uprev_Shared_BRAM_data_in'}},'Xilinx'=>{'jtaghwcosim'=>{'non_memory_mapped_port'=>'uprev_Shared_BRAM_data_in'},'xdspkit'=>{'non_memory_mapped_port'=>'uprev_Shared_BRAM_data_in'}}}
  kestfilt_60mhz_nyq2_dout1_0_data_out : xbsIndex_r4/Gateway In  gui_display_data_type=Fixed-point  arith_type=Unsigned  n_bits=64  bin_pt=0  preci_type=Single  exp_width=8  frac_width=24  quantization=Truncate  overflow=Wrap  period=sample_rate  dbl_ovrd=off  timing_constraint=None  locs_specified=off  LOCs={}  UseAsADC=off  ADCChannel='1'  inherit_from_input=off  hdl_port=on  block_type=gatewayin
      settings: xl_area=[0, 0, 0, 0, 0, 0, 0]
  kestfilt_60mhz_nyq2_dout1_0_we : xbsIndex_r4/Gateway Out  inherit_from_input=off  hdl_port=on  timing_constraint=None  locs_specified=off  LOCs={'A14'}  UseAsDAC=off  DACChannel='1'  block_type=gatewayout
      settings: infoedit="Gateway out block.  Converts Xilinx fixed point inputs into ouputs of type Simulink integer, double, or fixed point.<P><P>Hardware notes:  In hardware these blocks become top level output ports or are discarded, depending on how they are configured."  xl_area=[0, 0, 0, 0, 0, 0, 0]
  mem : Subsystem
  munge_in : Subsystem  AncestorBlock=casper_library_flow_control/munge  mask(munge){divisions=2, div_size=[32 32], order=[1  0], arith_type_out=Unsigned, bin_pt_out=0}
      mask prompts: divisions "Number of divisions"; div_size "Division size (bits)"; order "Division packing order"; arith_type_out "Output arithmetic type"; bin_pt_out "Output binary point"
      mask help: Splits an input bus into the specified number of divisions and then recombines them in the order specified (most significant division = 0,least = number divisions-1)
      mask init:
      | munge_init(gcb, ...
      |     'divisions', divisions, ...
      |     'div_size', div_size, ...
      |     'order', order, ...
      |     'arith_type_out', arith_type_out, ...
      |     'bin_pt_out', bin_pt_out);
      settings: AttributesFormatString=|
      | split:[32 32]
      | join:[1 0]
      | Unsigned [64,0]
      mask TypeOptions arith_type_out: Unsigned | Signed  (2's comp) | Floating-point
  munge_out : Subsystem  AncestorBlock=casper_library_flow_control/munge  mask(munge){divisions=2, div_size=[32 32], order=[1  0], arith_type_out=Unsigned, bin_pt_out=0}
      mask prompts: divisions "Number of divisions"; div_size "Division size (bits)"; order "Division packing order"; arith_type_out "Output arithmetic type"; bin_pt_out "Output binary point"
      mask help: Splits an input bus into the specified number of divisions and then recombines them in the order specified (most significant division = 0,least = number divisions-1)
      mask init:
      | munge_init(gcb, ...
      |     'divisions', divisions, ...
      |     'div_size', div_size, ...
      |     'order', order, ...
      |     'arith_type_out', arith_type_out, ...
      |     'bin_pt_out', bin_pt_out);
      settings: AttributesFormatString=|
      | split:[32 32]
      | join:[1 0]
      | Unsigned [64,0]
      mask TypeOptions arith_type_out: Unsigned | Signed  (2's comp) | Floating-point
  data_out : Outport
  wires:
  munge_in/1(dout) -> convert_din1/1
  munge_out/1(dout) -> data_out/1
  we/1 -> convert_we/1
  addr/1 -> calc_add/1(in)
  mem/1(Out1) -> kestfilt_60mhz_nyq2_dout1_0_data_out/1
  kestfilt_60mhz_nyq2_dout1_0_data_out/1 -> munge_out/1(din)
  convert_we/1 -> kestfilt_60mhz_nyq2_dout1_0_we/1
  kestfilt_60mhz_nyq2_dout1_0_addr/1 -> mem/1(In1)
  kestfilt_60mhz_nyq2_dout1_0_data_in/1 -> mem/2(In2)
  kestfilt_60mhz_nyq2_dout1_0_we/1 -> mem/3(In3)
  calc_add/1(out) -> convert_addr/1
  data_in/1 -> munge_in/1(din)
  convert_din1/1 -> kestfilt_60mhz_nyq2_dout1_0_data_in/1
  convert_addr/1 -> kestfilt_60mhz_nyq2_dout1_0_addr/1

== system kestfilt_2048ch_60mhz/dout2_0 ==
  addr : Inport
  data_in : Inport  Port=2
  we : Inport  Port=3
  calc_add : Subsystem  mask{data_width=64, addr_width=11, sample_rate=sample_rate}
      mask prompts: data_width "data width"; addr_width "address width"; sample_rate "sample rate"
  convert_addr : xbsIndex_r4/Convert  gui_display_data_type=Fixed-point  arith_type=Unsigned  n_bits=addr_width  bin_pt=0  float_type=Single  exp_bits=8  fraction_bits=24  quantization=Truncate  overflow=Wrap  en=off  latency=0  dbl_ovrd=off  pipeline=off  block_type=convert
      settings: xl_area=[0, 0, 0, 0, 0, 0, 0]
  convert_din1 : xbsIndex_r4/Convert  gui_display_data_type=Fixed-point  arith_type=Unsigned  n_bits=64  bin_pt=0  float_type=Single  exp_bits=8  fraction_bits=24  quantization=Truncate  overflow=Wrap  en=off  latency=0  dbl_ovrd=off  pipeline=off  block_type=convert
      settings: xl_area=[0, 0, 0, 0, 0, 0, 0]
  convert_we : xbsIndex_r4/Convert  gui_display_data_type=Fixed-point  arith_type=Unsigned  n_bits=1  bin_pt=0  float_type=Single  exp_bits=8  fraction_bits=24  quantization=Truncate  overflow=Wrap  en=off  latency=0  dbl_ovrd=off  pipeline=off  block_type=convert
      settings: xl_area=[0, 0, 0, 0, 0, 0, 0]
  kestfilt_60mhz_nyq2_dout2_0_addr : xbsIndex_r4/Gateway Out  inherit_from_input=off  hdl_port=on  timing_constraint=None  locs_specified=off  LOCs={'A5','B9','A9','C1','A3','G6','E9','A6','A7','A8','B8','B1','B3','D9','B5','B4','B6','C2'}  UseAsDAC=off  DACChannel='1'  block_type=gatewayout
      settings: infoedit="Gateway out block.  Converts Xilinx fixed point inputs into ouputs of type Simulink integer, double, or fixed point.<P><P>Hardware notes:  In hardware these blocks become top level output ports or are discarded, depending on how they are configured."  xl_area=[0, 0, 0, 0, 0, 0, 0]  sginterface={'Nallatech'=>{'xdspkit'=>{'non_memory_mapped_port'=>'uprev_Shared_BRAM_addr'}},'Xilinx'=>{'jtaghwcosim'=>{'non_memory_mapped_port'=>'uprev_Shared_BRAM_addr'},'xdspkit'=>{'non_memory_mapped_port'=>'uprev_Shared_BRAM_addr'}}}
  kestfilt_60mhz_nyq2_dout2_0_data_in : xbsIndex_r4/Gateway Out  inherit_from_input=off  hdl_port=on  timing_constraint=None  locs_specified=off  LOCs={'B21','B22','A22','B23','B19','C19','A20','A21','A23','B24','A24','A25','E18','D18','C18','B18'}  UseAsDAC=off  DACChannel='1'  block_type=gatewayout
      settings: infoedit="Gateway out block.  Converts Xilinx fixed point inputs into ouputs of type Simulink integer, double, or fixed point.<P><P>Hardware notes:  In hardware these blocks become top level output ports or are discarded, depending on how they are configured."  xl_area=[0, 0, 0, 0, 0, 0, 0]  sginterface={'Nallatech'=>{'xdspkit'=>{'non_memory_mapped_port'=>'uprev_Shared_BRAM_data_in'}},'Xilinx'=>{'jtaghwcosim'=>{'non_memory_mapped_port'=>'uprev_Shared_BRAM_data_in'},'xdspkit'=>{'non_memory_mapped_port'=>'uprev_Shared_BRAM_data_in'}}}
  kestfilt_60mhz_nyq2_dout2_0_data_out : xbsIndex_r4/Gateway In  gui_display_data_type=Fixed-point  arith_type=Unsigned  n_bits=64  bin_pt=0  preci_type=Single  exp_width=8  frac_width=24  quantization=Truncate  overflow=Wrap  period=sample_rate  dbl_ovrd=off  timing_constraint=None  locs_specified=off  LOCs={}  UseAsADC=off  ADCChannel='1'  inherit_from_input=off  hdl_port=on  block_type=gatewayin
      settings: xl_area=[0, 0, 0, 0, 0, 0, 0]
  kestfilt_60mhz_nyq2_dout2_0_we : xbsIndex_r4/Gateway Out  inherit_from_input=off  hdl_port=on  timing_constraint=None  locs_specified=off  LOCs={'A14'}  UseAsDAC=off  DACChannel='1'  block_type=gatewayout
      settings: infoedit="Gateway out block.  Converts Xilinx fixed point inputs into ouputs of type Simulink integer, double, or fixed point.<P><P>Hardware notes:  In hardware these blocks become top level output ports or are discarded, depending on how they are configured."  xl_area=[0, 0, 0, 0, 0, 0, 0]
  mem : Subsystem
  munge_in : Subsystem  AncestorBlock=casper_library_flow_control/munge  mask(munge){divisions=2, div_size=[32 32], order=[1  0], arith_type_out=Unsigned, bin_pt_out=0}
      mask prompts: divisions "Number of divisions"; div_size "Division size (bits)"; order "Division packing order"; arith_type_out "Output arithmetic type"; bin_pt_out "Output binary point"
      mask help: Splits an input bus into the specified number of divisions and then recombines them in the order specified (most significant division = 0,least = number divisions-1)
      mask init:
      | munge_init(gcb, ...
      |     'divisions', divisions, ...
      |     'div_size', div_size, ...
      |     'order', order, ...
      |     'arith_type_out', arith_type_out, ...
      |     'bin_pt_out', bin_pt_out);
      settings: AttributesFormatString=|
      | split:[32 32]
      | join:[1 0]
      | Unsigned [64,0]
      mask TypeOptions arith_type_out: Unsigned | Signed  (2's comp) | Floating-point
  munge_out : Subsystem  AncestorBlock=casper_library_flow_control/munge  mask(munge){divisions=2, div_size=[32 32], order=[1  0], arith_type_out=Unsigned, bin_pt_out=0}
      mask prompts: divisions "Number of divisions"; div_size "Division size (bits)"; order "Division packing order"; arith_type_out "Output arithmetic type"; bin_pt_out "Output binary point"
      mask help: Splits an input bus into the specified number of divisions and then recombines them in the order specified (most significant division = 0,least = number divisions-1)
      mask init:
      | munge_init(gcb, ...
      |     'divisions', divisions, ...
      |     'div_size', div_size, ...
      |     'order', order, ...
      |     'arith_type_out', arith_type_out, ...
      |     'bin_pt_out', bin_pt_out);
      settings: AttributesFormatString=|
      | split:[32 32]
      | join:[1 0]
      | Unsigned [64,0]
      mask TypeOptions arith_type_out: Unsigned | Signed  (2's comp) | Floating-point
  data_out : Outport
  wires:
  convert_addr/1 -> kestfilt_60mhz_nyq2_dout2_0_addr/1
  convert_din1/1 -> kestfilt_60mhz_nyq2_dout2_0_data_in/1
  data_in/1 -> munge_in/1(din)
  calc_add/1(out) -> convert_addr/1
  kestfilt_60mhz_nyq2_dout2_0_we/1 -> mem/3(In3)
  kestfilt_60mhz_nyq2_dout2_0_data_in/1 -> mem/2(In2)
  kestfilt_60mhz_nyq2_dout2_0_addr/1 -> mem/1(In1)
  convert_we/1 -> kestfilt_60mhz_nyq2_dout2_0_we/1
  kestfilt_60mhz_nyq2_dout2_0_data_out/1 -> munge_out/1(din)
  mem/1(Out1) -> kestfilt_60mhz_nyq2_dout2_0_data_out/1
  addr/1 -> calc_add/1(in)
  we/1 -> convert_we/1
  munge_out/1(dout) -> data_out/1
  munge_in/1(dout) -> convert_din1/1
